simulink model "hardware"  (R2023a)
settings: Solver=FixedStepDiscrete  StartTime=0.0  StopTime=10  FixedStep=0.001  RelTol=1e-3  EnableMultiTasking=on
values from neighbouring files (symbols this model uses):
  T = 0.001    [Config.mat]    (also in parameters_calculate.m; pendubot_dynamics.m = 0.1)
undefined symbols (not defined in the file or in its folder): HIL
libraries: quarc_library x3
settings Model: SimulationMode=external  ExtModeTrigType=signal  ExtModeTrigDuration=10000  ExtModeTrigDirection=either  ExtModeTrigLevel=0.500000  Creator=colegiusto  LastModifiedBy=tianyi_chen
settings SolverCC: PositivePriorityOrder=on
settings RTWCC: Description=QUARC Win64 Target Using Toolchain  SystemTargetFile=quarc_win64.tlc  Toolchain=QUARC win64 | nmake (64-bit Windows)  BuildConfiguration=Faster Runs
settings STFCustomTargetCC: TargetLangStandard=C89/C90 (ANSI)  SystemTargetFile=quarc_win64.tlc
settings GRTTargetCC: TargetLangStandard=C89/C90 (ANSI)  ParMdlRefBuildCompliant=off  CompOptLevelCompliant=off  CombineOutputUpdateFcns=off  MatFileLogging=off  CPPClassGenCompliant=off  GRTInterface=on  ExtMode=on  ExtModeMexFile=quarc_comm

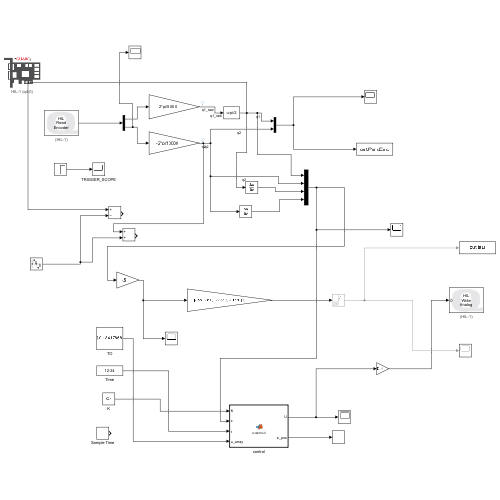
[thumbnail: Simulink's stored preview of the top-level diagram]
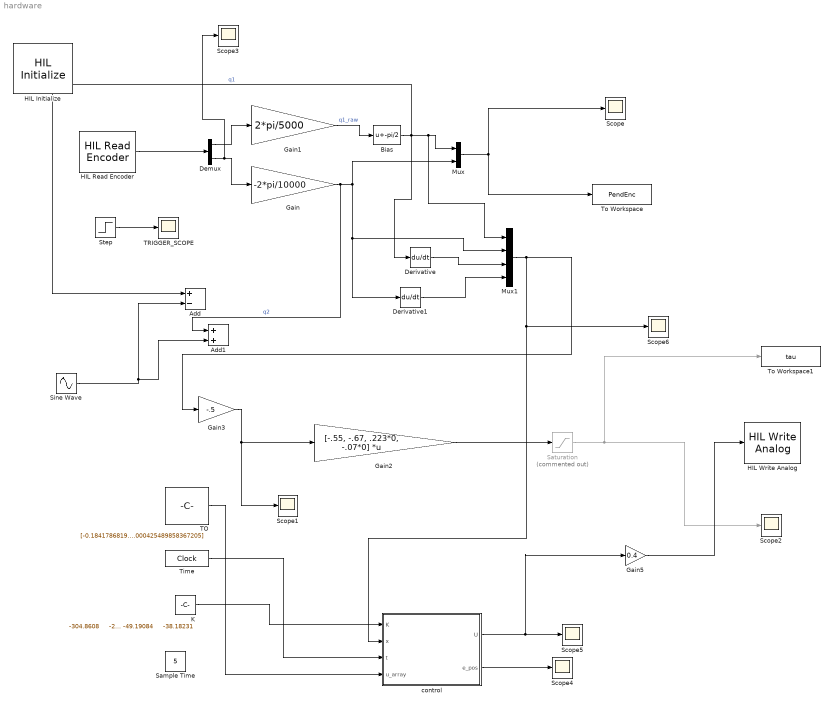
== system hardware ==
  Add : Sum  Inputs=+-
  Add1 : Sum
  Bias : Bias  Bias=-pi/2  SaturateOnIntegerOverflow=off
  Demux : Demux  Outputs=2
  Derivative : Derivative  CoefficientInTFapproximation=0.05
  Derivative1 : Derivative  CoefficientInTFapproximation=0.05
  Gain : Gain  Gain=-2*pi/10000
  Gain1 : Gain  Gain=2*pi/5000
  Gain2 : Gain  Gain=[-.55, -.67, .223*0, -.07*0]  Multiplication=Matrix(K*u)
  Gain3 : Gain  Gain=-.5
  Gain5 : Gain  Gain=0.4
  HIL Initialize : quarc_library/Data Acquisition/Generic/Configuration/HIL Initialize  object_name=HIL-1  board_type=q4  board_number=0  board_options=""  exclusive=off  active=on  hardware_clocks=[0:1]  clock_modes=[0 0]  initial_clock_frequencies=[]  set_clock_params_at_start=on  set_clock_params_at_switch_in=off  set_clock_frequencies_at_start=off  set_clock_frequencies_at_switch_in=off  analog_input_channels=[0:3]  analog_input_configurations=[]  analog_input_maximums=10  analog_input_minimums=-10  set_analog_input_params_at_start=off  set_analog_input_params_at_switch_in=off  analog_output_channels=[0:3]  analog_output_maximums=[10]  analog_output_minimums=[-10]  initial_analog_outputs=[0]  final_analog_outputs=[0]  watchdog_analog_outputs=0  set_analog_output_params_at_start=on  set_analog_output_params_at_switch_in=off  set_analog_outputs_at_start=on  set_analog_outputs_at_switch_in=off  set_analog_outputs_at_terminate=on  set_analog_outputs_at_switch_out=off  set_analog_outputs_on_watchdog=off  digital_input_channels=[]  digital_output_channels=[]  digital_output_configuration=[]  initial_digital_outputs=[1]  final_digital_outputs=[1]  watchdog_digital_outputs=[2]  set_digital_output_params_at_start=off  set_digital_output_params_at_switch_in=off  set_digital_outputs_at_start=on  set_digital_outputs_at_switch_in=off  set_digital_outputs_at_terminate=on  set_digital_outputs_at_switch_out=off  set_digital_outputs_on_watchdog=off  encoder_channels=[0:3]  quadrature=[4]  encoder_filter_frequency=(1/60e-9)/1  initial_encoder_counts=[0]  set_encoder_params_at_start=on  set_encoder_params_at_switch_in=off  set_encoder_counts_at_start=on  set_encoder_counts_at_switch_in=off  pwm_channels=[]  pwm_modes=[0]  pwm_frequency=(1/60e-9)/1024  pwm_configuration=[]  pwm_alignment=[]  pwm_polarity=[]  pwm_leading_deadband=[]  pwm_trailing_deadband=[]  initial_pwm_outputs=[0]  final_pwm_outputs=[0]  watchdog_pwm_outputs=[]  set_pwm_params_at_start=on  set_pwm_params_at_switch_in=off  set_pwm_outputs_at_start=on  set_pwm_outputs_at_switch_in=off  set_pwm_outputs_at_terminate=on  set_pwm_outputs_at_switch_out=off  set_pwm_outputs_on_watchdog=off  other_output_channels=[]  initial_other_outputs=[]  final_other_outputs=[]  watchdog_other_outputs=[]  set_other_outputs_at_start=off  set_other_outputs_at_switch_in=off  set_other_outputs_at_terminate=off  set_other_outputs_at_switch_out=off  set_other_outputs_on_watchdog=off
  HIL Read Encoder : quarc_library/Data Acquisition/Generic/Immediate I//O/HIL Read Encoder  object_name=HIL-1  channels=[0:1]  sample_time=0.001  active=on  vector_output=on  data_type_mode=Inherit via back propagation  data_type=double
  HIL Write Analog : quarc_library/Data Acquisition/Generic/Immediate I//O/HIL Write Analog  object_name=HIL-1  channels=0  sample_time=0.001  active=off  vector_input=off
  K : Constant  Value="-304.8608     -290.7186     -49.19084     -38.18231"
  Mux : Mux  Inputs=2
  Mux1 : Mux
  Sample Time : Constant  Value=5
  Saturation : Saturate  Commented=on  UpperLimit=2  LowerLimit=-2
  Scope{,1..6} (7 alike) : Scope
  Sine Wave : Sin  Amplitude=2  Bias=.05  Frequency=5  SampleTime=0.001
  Step : Step  Time=0.001  SampleTime=0
  TO : Constant  Value=[-0.18417868194945 -0.226841825144858 -0.290388060159798 -0.314153466552654 -0.308261482997459 -0.286417490775861 -0.262301789640817 -0.246233380730292 -0.244248621928876 -0.259477215448114 -0.293934669646237 -0.348894125876957 -0.423403657565455 -0.511677310377363 -0.601627977133467 -0.676430918179053 -0.718422561822155 -0.712511019574875 -0.647970404116223 -0.519951509047282 -0.331896127027282 -0.0970879861599679 0.163144637027244 0.425149605488482 0.672247343663993 0.903249670683672 1.33006753252278 1.92855033896873 2.28336863228776 2.413587860541 2.47036827661979 2.4462307006074 2.33428711218315 2.13811525682842 1.87509408092419 1.57374332189617 1.2672386165449 0.985534643909603 0.748579949179877 0.563568993492329 0.426667537303137 0.32811793624088 0.257203155351971 0.205159287150929 0.165872479811284 0.135358324477574 0.111102565269 0.0915312815165523 0.0755502355047744 0.0624124996816075 0.0515923634781224 0.0426346750247846 0.0352394915399667 0.0291145292033053 0.0240408799502026 0.0198409473221717 0.0163541749387641 0.0135205448952492 0.011162838300063 0.00922450988708832 0.00760224958330253 0.0062581258388429 0.00516281356975343 0.0042587214304924 0.00352050342775851 0.00290094446872515 0.00238699039421767 0.00197507435193779 0.00160776213081181 0.00132880259640431 0.00109368035298884 0.000911230170358577 0.000735757966109276 0.000604302503621639 0.000484728064077338 0.000404041824444067 0.000321176650142435 0.000258991116225125 0.000182976572813051 0.000137441784731778 0.00010371344554284 7.12917259653379e-05 2.6522007724356e-05 -8.23106735140368e-07 -2.66060341439223e-05 -6.45125251826262e-05 -9.64651593982654e-05 -0.000130835391011356 -0.000179221234127311 -0.000210599518358178 -0.000255655296496385 -0.00027970724721437 -0.000316119690057687 -0.000329268699052391 -0.000322904148534204 -0.000301428279027518 -0.000222012835024778 -5.68396177541383e-05 0.000236410682607981 0.000425489858367205]
  TRIGGER_SCOPE : Scope
  Time : DigitalClock  SampleTime=T
  To Workspace : ToWorkspace  VariableName=PendEnc  SaveFormat=Structure With Time  SampleTime=-1
  To Workspace1 : ToWorkspace  VariableName=tau  SaveFormat=Structure With Time  SampleTime=-1
  control : MATLAB Function  TreatAsAtomicUnit=on
  wires:
  Sine Wave/1 -> Add/2, Add1/2
  Step/1 -> TRIGGER_SCOPE/1
  HIL Read Encoder/1 -> Demux/1
  Demux/1 -> Gain1/1
  Demux/2 -> Scope3/1, Gain/1
  Gain/1 -> Add1/1, Mux1/2, Derivative1/1, Mux/2  "q2"
  Mux/1 -> Scope/1, To Workspace/1
  Derivative/1 -> Mux1/3
  Derivative1/1 -> Mux1/4
  Gain2/1 -> Saturation/1
  Saturation/1 -> To Workspace1/1, Scope2/1
  Gain3/1 -> Scope1/1, Gain2/1
  Gain1/1 -> Bias/1  "q1_raw"
  Mux1/1 -> Gain3/1, control/2(x), Scope6/1
  K/1 -> control/1(K)
  TO/1 -> control/4(u_array)
  Time/1 -> control/3(t)
  control/2(e_pos) -> Scope4/1
  control/1(U) -> Gain5/1, Scope5/1
  Bias/1 -> Derivative/1, Add/1, Mux1/1, Mux/1  "q1"
  Gain5/1 -> HIL Write Analog/1

== matlab function hardware/control ==
  data: K input; x input; t input; u_array input; U output size=1; e_pos output
function [U, e_pos] = control(K, x, t, u_array)
    % x(1) = x(1)-pi/2;
    
    xF=[pi/2;0;0;0];u_max=3;
    persistent lqr_engaged
    % Reset the memory if it's the start of simulation (t=0)
    % or if the variable hasn't been created yet.
    if isempty(lqr_engaged) || t == 0
        lqr_engaged = false;
    end

    x(3:4) = vel_estimator(x(1:2));
    % 1. Calculate Error
    error = x - xF;
    % 2. Define Switching Condition
    % Switch to LQR if position is close AND velocity is manageable
    e_pos = atan2(sin(error(1:2)), cos(error(1:2)));
    pos_err = norm(e_pos);
    e_vel = error(3:4);
    vel_err = norm(e_vel);
    %disp(error)
    u=1;
    % Thresholds: e.g., within 0.3 rad (approx 17 deg) and moving slowly
    if ((pos_err >= 0.4) || (vel_err >= 10.0)) && (lqr_engaged == false)
        % --- SWING UP MODE (Trajectory Playback) ---
        mode = 0;
        u=interp1([0:1:99],u_array, ((t+0.001)/3.001) * 100, 'linear', 'extrap');
        %disp('TO Activated');
    else
        lqr_engaged = true;
        % --- LQR MODE ---
        mode = 1;
        x_error = [e_pos; e_vel];
        x_error = x_error(1:4, 1);
        K= K';
        v = -K(1,1:4)*x_error;
        u = inverse_dynamics_pfl(x,v);
        u = u(1);
        %disp('PFL-LQR Activated');
    end
    % 3. Saturation (Physical Limits)
    U = max(min(u, u_max), -u_max);
end

function dq = vel_estimator(q)
% q  : [q1; q2] (rad)
% dq : [dq1; dq2] estimated velocities (rad/s)

% === Parameters ===
Ts    = 0.001;    % sample time (s) - match your HIL sample time
alpha = 0.95;     % smoothing factor (0<alpha<1)

persistent q_prev dq_prev
if isempty(q_prev)
    q_prev = q;
    dq_prev = [0; 0];
end

% raw finite-difference derivative
dq_raw = (q - q_prev) / Ts;

% filtered derivative ("dirty derivative")
dq = alpha * dq_prev + (1-alpha) * dq_raw;

% update memory
q_prev = q;
dq_prev = dq;
end


function tau = inverse_dynamics_pfl(x, v)
    % Unpack
    % q1 = x(1); q2 = x(2); dq1 = x(3); dq2 = x(4);
    
    [D, H, Phi] = get_matrices(x);
    d11 = D(1,1); d12 = D(1,2);
    d21 = D(2,1); d22 = D(2,2);
    h1 = H(1); h2 = H(2);
    phi1 = Phi(1); phi2 = Phi(2);
    
    % From PFL derivation (Collocated Linearization):
    % tau = M_bar * v + N_bar
    
    % M_bar = d11 - d12*inv(d22)*d21
    m_bar = d11 - (d12 * d21 / d22);
    
    % N_bar = (h1 + phi1) - d12*inv(d22)*(h2 + phi2)
    n_bar = (h1 + phi1) - (d12 / d22) * (h2 + phi2);
    
    tau = m_bar * v + n_bar;
end

% --- Standard Matrices Helper ---
function [D, H, Phi] = get_matrices(x)
    q1 = x(1); q2 = x(2); dq1 = x(3); dq2 = x(4);
    
    g   = 9.81;
    Th1 = 3.08e-2; Th2 = 1.06e-2; Th3 = 9.5e-3;
    Th4 = 2.087e-1; Th5 = 6.3e-2;
    
    c2 = cos(q2); s2 = sin(q2);
    c1 = cos(q1); c12 = cos(q1+q2);

    D = [Th1 + Th2 + 2*Th3*c2,  Th2 + Th3*c2;
         Th2 + Th3*c2,          Th2];
     
    h_term = Th3 * s2;
    H = [-h_term * dq2 * (2*dq1 + dq2);
          h_term * dq1^2];
      
    Phi = [Th4*g*c1 + Th5*g*c12;
           Th5*g*c12];
end

% function u=u_t_TO(u_array, t)
% %display(t);
% u=interp1([0:1:99],u_array, t/3 *100, 'linear', 'extrap');
% end
